simulink model "SixDOFSim"  (R2020b)
settings: Solver=VariableStepAuto  StartTime=0.0  StopTime=80  RelTol=1e-3
values from neighbouring files (symbols this model uses):
  A = sys_ol.A    [cost_condition_number.m]    (also in cost_coupling_control.m; cost_filter.m; coupling_control_scratch.m = sys.A; coupling_control_scratch2.m = sys.A)
  B = sys_ol.B    [cost_condition_number.m]    (also in cost_coupling_control.m; cost_filter.m; coupling_control_scratch.m = sys.B; coupling_control_scratch2.m = sys.B)
  C_tilde = zeros(size(C,1), size(A,1))    [SixDOFModel.m]    (also in cost_condition_number.m = struct_cond.C_tilde; cost_coupling_control.m = struct_cond.C_tilde; cost_filter.m = struct_cond.C_tilde; coupling_controller.m = T*C_resort)
  deltaX_init = Tx\deltaX_init    [SixDOFModel.m]    (also in coupling_controller_main.m = X_init-X_ap_simulink)
  eta_max = 15*pi/180    (= 0.261799387799)    [SixDOFModel.m]    (also in coupling_controller_main.m = 0.174532925199; load_messung_one_massmodel.m = 0.174532925199)
  eta_min = - 30*pi/180    (= -0.523598775598)    [SixDOFModel.m]    (also in coupling_controller_main.m = -0.436332312999; load_messung_one_massmodel.m = -0.436332312999)
  F = real(F)    [coupling_control_scratch.m]    (also in coupling_control_scratch2.m; coupling_controller.m = Kopt{end}; coupling_controller_main.m = -inv(C*(Ak\B)); coupling_controller_philipp.m = -inv(C*(Ak\B)))
  F_mod = F_ent(:,1:p/2)    [SixDOFModel.m]    (also in coupling_controller_main.m = F1*Q_mod; coupling_controller_philipp.m = F1*Q_mod; script_kein_theta_verk.m = F1*Q_mod)
  K_coupling = inv(Dstar)*compR    [SixDOFModel.m]    (also in coupling_controller_main.m = Kopt{1}; coupling_controller_philipp.m = Kopt{1}; script_kein_theta_verk.m = Kopt{1})
  latlon_init = [0;0]    [SixDOFModel.m]    (also in create_multi_model.m)
  m = i-1    [coupling_control_scratch.m]    (also in coupling_control_scratch2.m; defineABC.m = size(B_1,2) + size(B_2,2); implicit_linmod.m = length(U_ap); initializeParameters.m = 120000)
  noise_weight = [10 10 10 1 1 1 1 1 10 10 10 10 1 1 1 1 1 10]'    [SixDOFModel.m]
  P_e_init_1 = [0;0;-h_init_1]    [SixDOFModel.m]    (also in create_multi_model.m)
  P_e_init_2 = [0;0;-h_init_2]    [SixDOFModel.m]    (also in create_multi_model.m)
  q = X(5)    [nonlinear_6DOF.m]    (also in normieren.m = size (C,1))
  r = 5    [coupling_controller.m]    (also in coupling_controller_main.m = 100; coupling_controller_philipp.m = 200; nonlinear_6DOF.m = X(6); polgebiet.m = a2)
  sigmaf_max = 20*pi/180    (= 0.349065850399)    [SixDOFModel.m]    (also in coupling_controller_main.m; load_messung_one_massmodel.m)
  sigmaf_min = 0.5*pi/180    (= 0.00872664625997)    [SixDOFModel.m]    (also in coupling_controller_main.m; load_messung_one_massmodel.m)
  Tu = eye(size(B,2))    [SixDOFModel.m]    (also in normieren.m = zeros(p,p))
  Tx = eye(n)    [SixDOFModel.m]    (also in normieren.m = diag([200 15 50 0.1 0.1 0.1 45*pi/180 45*pi/180 10000 200 15)
  Ty = eye(size(C,1))    [SixDOFModel.m]    (also in normieren.m = zeros(q,q))
  U_ap = Tu\U_ap    [SixDOFModel.m]    (also in coupling_controller_main.m = AP(1,1).U_ap; create_multi_model.m = [U_ap_1;U_ap_2]; fsolve_trim.m = ap(11:14); trimValues.m = Z_ap(11:14))
  W_ap = W_ap(1:4)    [SixDOFModel.m]    (also in coupling_controller_philipp.m = (C*X_ap_simulink)')
  X_ap = [X_ap_1;X_ap_2]    [SixDOFModel.m]    (also in coupling_controller_main.m = AP(1,1).X_ap; create_multi_model.m; fsolve_trim.m = ap(1:10); trimValues.m = Z_ap(1:10))
  X_ap_simulink = Tx\X_ap_simulink    [SixDOFModel.m]    (also in coupling_controller_main.m = AP(1,1).X_ap_simulink; create_multi_model.m = [X_ap(1:8);X_ap(10);X_ap(11:18);X_ap(20)])
  X_init = Tx\X_init    [SixDOFModel.m]    (also in cost_coupling_control.m = struct_cond.X_init; cost_filter.m = struct_cond.X_init; coupling_controller_main.m = X_ap_simulink; create_multi_model.m = [X_init_1; X_init_2])
  xi_max = 25*pi/180    (= 0.436332312999)    [SixDOFModel.m]    (also in coupling_controller_main.m; load_messung_one_massmodel.m)
  xi_min = - xi_max    (= -0.436332312999)    [SixDOFModel.m]    (also in coupling_controller_main.m; load_messung_one_massmodel.m)
  zita_max = 30*pi/180    (= 0.523598775598)    [SixDOFModel.m]    (also in coupling_controller_main.m; load_messung_one_massmodel.m)
  zita_min = - zita_max    (= -0.523598775598)    [SixDOFModel.m]    (also in coupling_controller_main.m; load_messung_one_massmodel.m)
undefined symbols (not defined in the file or in its folder): Earth, globalParameters, Light, MIL, WGS84
libraries: aerolibfltsims x24, aerolibtransform2 x4, aerolibwind2 x4, simulink x3, shared6dof x1, aerolibanim x1
(part 1 of 3)
settings Model: Creator=teteu  LastModifiedBy=Markus
settings SolverCC: ZeroCrossAlgorithm=Adaptive
settings DebuggingCC: IgnoredZcDiagnostic=none  UnderSpecifiedDimensionMsg=warning

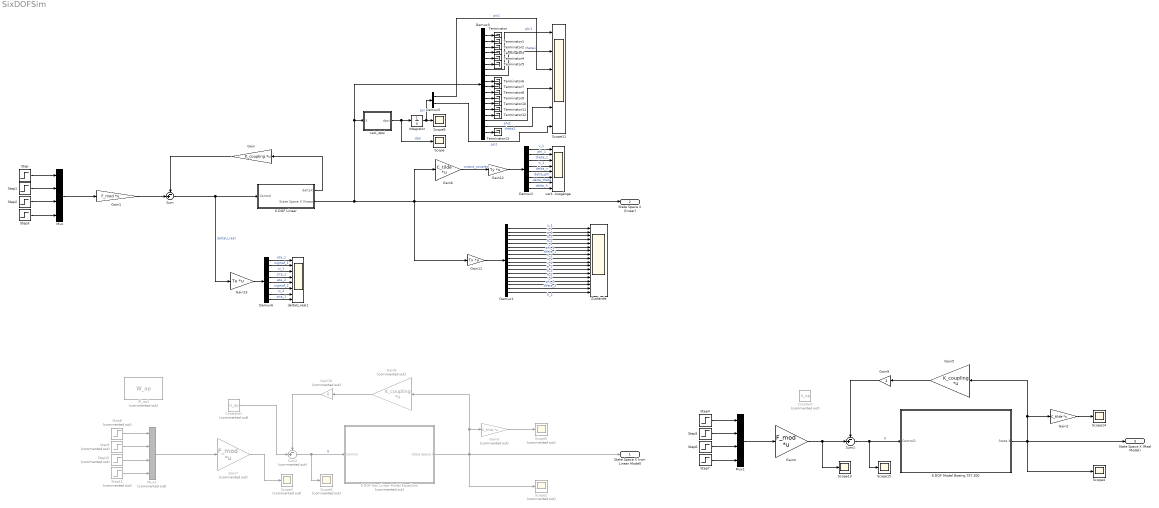
== system SixDOFSim ==
  6 DOF Linear : Subsystem
  6 DOF Model Boeing 757 200 : Subsystem
      mask Display: image('Eastern_Airlines_Boeing_757-225_N523EA_March_1990_DCW_4974892113-624x422.jpg'); % Use "Edit Image" on toolstrip to change.
  6 DOF Non Linear Model Equations : Subsystem  Commented=on
      mask Display: image('491461_1_En_8_Fig2_HTML.png');
  Constant : Constant  Commented=on  Value=U_ap
  Constant1 : Constant  Commented=on  Value=U_ap
  Demux1 : Demux  Outputs=18
  Demux2 : Demux  Outputs=8
  Demux3 : Demux  Outputs=18
  Demux5 : Demux  Outputs=2
  Demux6 : Demux  Outputs=8
  Gain : Gain  Gain=K_coupling  Multiplication=Matrix(K*u)
  Gain1 : Gain  Gain=F_mod  Multiplication=Matrix(K*u)
  Gain10 : Gain  Commented=on  Gain=0
  Gain11 : Gain  Gain=Tx  Multiplication=Matrix(K*u)
  Gain12 : Gain  Gain=Ty  Multiplication=Matrix(K*u)
  Gain13 : Gain  Gain=Tu  Multiplication=Matrix(K*u)
  Gain2 : Gain  Gain=C_tilde  Multiplication=Matrix(K*u)
  Gain3 : Gain  Commented=on  Gain=C_tilde  Multiplication=Matrix(K*u)
  Gain4 : Gain  Gain=F_mod  Multiplication=Matrix(K*u)
  Gain5 : Gain  Gain=K_coupling  Multiplication=Matrix(K*u)
  Gain6 : Gain  Gain=C_tilde  Multiplication=Matrix(K*u)
  Gain7 : Gain  Commented=on  Gain=F_mod  Multiplication=Matrix(K*u)
  Gain8 : Gain  Commented=on  Gain=K_coupling  Multiplication=Matrix(K*u)
  Gain9 : Gain
  Integrator : Integrator
  Mux : Mux
  Mux1 : Mux
  Mux2 : Mux  Commented=on
  Scope{,4,9,13..15} (6 alike) : Scope
  Scope11 : Scope  NumInputPorts=6
  Scope{2..3,5..6} (4 alike) : Scope  Commented=on
  Step{,1..3,5} (5 alike) : Step  Time=10  After=0  SampleTime=0
  Step10 : Step  Commented=on  Time=10  After=0  SampleTime=0
  Step11 : Step  Commented=on  Time=10  SampleTime=0
  Step4 : Step  Time=0  After=0  SampleTime=0
  Step6 : Step  Time=0  After=-0.0734  SampleTime=0
  Step7 : Step  Time=0  After=5000  SampleTime=0
  Step8 : Step  Commented=on  Time=10  After=0  SampleTime=0
  Step9 : Step  Commented=on  Time=10  After=0  SampleTime=0
  Sum : Sum  Inputs=-+|
  Sum1 : Sum  Inputs=-+|
  Sum2 : Sum  Commented=on  Inputs=-+|
  Terminator{,1..13} (14 alike) : Terminator
  W_ap1 : Constant  Commented=on  Value=W_ap
  Zustände : Scope  NumInputPorts=18
  calc_dpsi : MATLAB Function  TreatAsAtomicUnit=on
  deltaU_real1 : Scope  NumInputPorts=8
  verk. Ausgänge : Scope  NumInputPorts=8
  State Space X (non Linear Model) : Outport
  State Space X (linear) : Outport  Port=2
  State Space X (Real Model) : Outport  Port=3
  wires:
  Gain/1 -> Sum/1
  6 DOF Non Linear Model Equations/1(State Space X) -> Gain8/1, Gain3/1, State Space X (non Linear Model)/1, Scope2/1
  Mux/1 -> Gain1/1
  Gain1/1 -> Sum/2
  6 DOF Linear/1(deltaX) -> Gain/1
  Gain3/1 -> Scope5/1
  Gain6/1 -> Gain12/1  "output_coupled"
  Sum2/1 -> Scope6/1, 6 DOF Non Linear Model Equations/1(Control)  "U"
  Gain8/1 -> Gain10/1
  Gain7/1 -> Scope3/1
  Mux2/1 -> Gain7/1
  Demux1/1 -> Zustände/1  "u_1"
  Demux1/2 -> Zustände/2  "v_1"
  Demux1/3 -> Zustände/3  "w_1"
  Demux1/4 -> Zustände/4  "p_1"
  Demux1/5 -> Zustände/5  "q_1"
  Demux1/6 -> Zustände/6  "r_1"
  Demux1/7 -> Zustände/7  "phi_1"
  Demux1/8 -> Zustände/8  "theta_1"
  Demux1/9 -> Zustände/9  "h_1"
  Demux1/10 -> Zustände/10  "u_2"
  Demux1/11 -> Zustände/11  "v_2"
  Demux1/12 -> Zustände/12  "w_2"
  Demux1/13 -> Zustände/13  "p_2"
  Demux1/14 -> Zustände/14  "q_2"
  Demux1/15 -> Zustände/15  "r_2"
  Demux1/16 -> Zustände/16  "phi_2"
  Demux2/8 -> verk. Ausgänge/8  "delta_h"
  Demux2/7 -> verk. Ausgänge/7  "delta_theta"
  Demux2/6 -> verk. Ausgänge/6  "delta_phi"
  Demux2/3 -> verk. Ausgänge/3  "theta_1"
  Demux2/2 -> verk. Ausgänge/2  "phi_1"
  Demux2/4 -> verk. Ausgänge/4  "h_1"
  Demux2/5 -> verk. Ausgänge/5  "delta_v"
  Demux2/1 -> verk. Ausgänge/1  "v_1"
  calc_dpsi/1(dpsi) -> Scope/1, Integrator/1  "dpsi"
  Integrator/1 -> Demux5/1, Scope9/1  "psi"
  Demux3/1 -> Terminator/1
  Demux3/2 -> Terminator1/1
  Demux3/3 -> Terminator2/1
  Demux3/4 -> Terminator3/1
  Demux3/5 -> Terminator4/1
  Demux3/6 -> Terminator5/1
  Demux3/7 -> Scope11/1  "phi1"
  Demux3/8 -> Scope11/2  "theta1"
  Demux3/10 -> Terminator7/1
  Demux3/11 -> Terminator8/1
  Demux3/12 -> Terminator9/1
  Demux3/13 -> Terminator10/1
  Demux3/14 -> Terminator11/1
  Demux3/16 -> Scope11/4  "phi2"
  Demux5/1 -> Scope11/3  "psi1"
  Demux5/2 -> Scope11/6  "psi2"
  6 DOF Linear/2(State Space X (linear)) -> Demux3/1, calc_dpsi/1(X), State Space X (linear)/1, Gain11/1, Gain6/1
  Demux1/18 -> Zustände/18  "h_2"
  Demux1/17 -> Zustände/17  "theta_2"
  Demux3/9 -> Terminator6/1
  Demux3/15 -> Terminator12/1
  Demux3/17 -> Scope11/5  "theta2"
  Demux3/18 -> Terminator13/1
  Step/1 -> Mux/1
  Step1/1 -> Mux/2
  Step2/1 -> Mux/3
  Step3/1 -> Mux/4
  Sum1/1 -> 6 DOF Model Boeing 757 200/1(Control1), Scope15/1  "U"
  Gain4/1 -> Sum1/2, Scope13/1
  6 DOF Model Boeing 757 200/1(State X) -> State Space X (Real Model)/1, Gain5/1, Gain2/1, Scope4/1
  Gain2/1 -> Scope14/1
  Gain5/1 -> Gain9/1
  Step7/1 -> Mux1/4
  Step6/1 -> Mux1/3
  Step4/1 -> Mux1/1
  Step5/1 -> Mux1/2
  Mux1/1 -> Gain4/1
  Step11/1 -> Mux2/4
  Step10/1 -> Mux2/3
  Step8/1 -> Mux2/1
  Step9/1 -> Mux2/2
  Gain9/1 -> Sum1/1
  Gain10/1 -> Sum2/1
  Constant1/1 -> Sum2/2
  Gain11/1 -> Demux1/1
  Gain12/1 -> Demux2/1
  Demux6/4 -> deltaU_real1/4  "zita_1"
  Demux6/3 -> deltaU_real1/3  "xi_1"
  Demux6/7 -> deltaU_real1/7  "xi_2"
  Demux6/6 -> deltaU_real1/6  "sigmaf_2"
  Demux6/1 -> deltaU_real1/1  "eta_1"
  Demux6/2 -> deltaU_real1/2  "sigmaf_1"
  Demux6/5 -> deltaU_real1/5  "eta_2"
  Sum/1 -> Gain13/1, 6 DOF Linear/1(Control)  "deltaU_real"
  Demux6/8 -> deltaU_real1/8  "zita_2"
  Gain13/1 -> Demux6/1

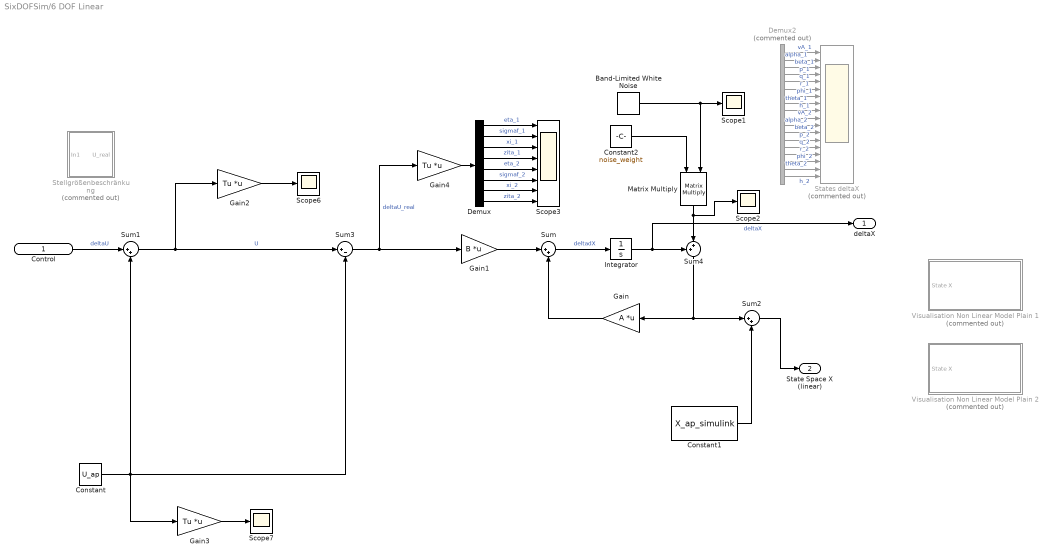
== system SixDOFSim/6 DOF Linear ==
  Control : Inport
  Band-Limited White Noise : simulink/Sources/Band-Limited White Noise  Cov=[0.0]  Ts=0.01  seed=[23341]
  Constant : Constant  Value=U_ap
  Constant1 : Constant  Value=X_ap_simulink
  Constant2 : Constant  Value=noise_weight
  Demux : Demux  Outputs=8
  Demux2 : Demux  Commented=on  Outputs=18
  Gain : Gain  Gain=A  Multiplication=Matrix(K*u)
  Gain1 : Gain  Gain=B  Multiplication=Matrix(K*u)
  Gain2 : Gain  Gain=Tu  Multiplication=Matrix(K*u)
  Gain3 : Gain  Gain=Tu  Multiplication=Matrix(K*u)
  Gain4 : Gain  Gain=Tu  Multiplication=Matrix(K*u)
  Integrator : Integrator  InitialCondition=deltaX_init
  Matrix Multiply : Product  Multiplication=Matrix(*)
  Scope{1..2,6..7} (4 alike) : Scope
  Scope3 : Scope  NumInputPorts=8
  States deltaX : Scope  Commented=on  NumInputPorts=18
  Stellgrößenbeschränkung : Subsystem  Commented=on
  Sum : Sum  Inputs=|++
  Sum1 : Sum  Inputs=|++
  Sum2 : Sum  Inputs=|++
  Sum3 : Sum  Inputs=|+-
  Sum4 : Sum  Inputs=++|
  Visualisation Non Linear Model Plain 1 : Subsystem  Commented=on
  Visualisation Non Linear Model Plain 2 : Subsystem  Commented=on
  deltaX : Outport
  State Space X (linear) : Outport  Port=2
  wires:
  Gain1/1 -> Sum/1
  Sum/1 -> Integrator/1  "deltadX"
  Gain/1 -> Sum/2
  Control/1 -> Sum1/1  "deltaU"
  Constant/1 -> Gain3/1, Sum1/2, Sum3/2
  Sum1/1 -> Sum3/1, Gain2/1  "U"
  Sum2/1 -> State Space X (linear)/1
  Constant1/1 -> Sum2/2
  Sum3/1 -> Gain4/1, Gain1/1  "deltaU_real"
  Demux/1 -> Scope3/1  "eta_1"
  Demux/2 -> Scope3/2  "sigmaf_1"
  Demux/3 -> Scope3/3  "xi_1"
  Demux/4 -> Scope3/4  "zita_1"
  Demux/5 -> Scope3/5  "eta_2"
  Demux/6 -> Scope3/6  "sigmaf_2"
  Demux/7 -> Scope3/7  "xi_2"
  Demux/8 -> Scope3/8  "zita_2"
  Demux2/9 -> States deltaX/9  "h_1"
  Demux2/13 -> States deltaX/13  "p_2"
  Demux2/6 -> States deltaX/6  "r_1"
  Demux2/15 -> States deltaX/15  "r_2"
  Demux2/18 -> States deltaX/18  "h_2"
  Demux2/14 -> States deltaX/14  "q_2"
  Demux2/8 -> States deltaX/8  "theta_1"
  Demux2/17 -> States deltaX/17  "theta_2"
  Demux2/11 -> States deltaX/11  "alpha_2"
  Demux2/2 -> States deltaX/2  "alpha_1"
  Demux2/3 -> States deltaX/3  "beta_1"
  Demux2/1 -> States deltaX/1  "vA_1"
  Demux2/16 -> States deltaX/16  "phi_2"
  Demux2/12 -> States deltaX/12  "beta_2"
  Demux2/4 -> States deltaX/4  "p_1"
  Demux2/7 -> States deltaX/7  "phi_1"
  Demux2/5 -> States deltaX/5  "q_1"
  Demux2/10 -> States deltaX/10  "vA_2"
  Integrator/1 -> deltaX/1, Sum4/1  "deltaX"
  Sum4/1 -> Sum2/1, Gain/1
  Band-Limited White Noise/1 -> Matrix Multiply/2, Scope1/1
  Constant2/1 -> Matrix Multiply/1
  Matrix Multiply/1 -> Sum4/2, Scope2/1
  Gain2/1 -> Scope6/1
  Gain3/1 -> Scope7/1
  Gain4/1 -> Demux/1

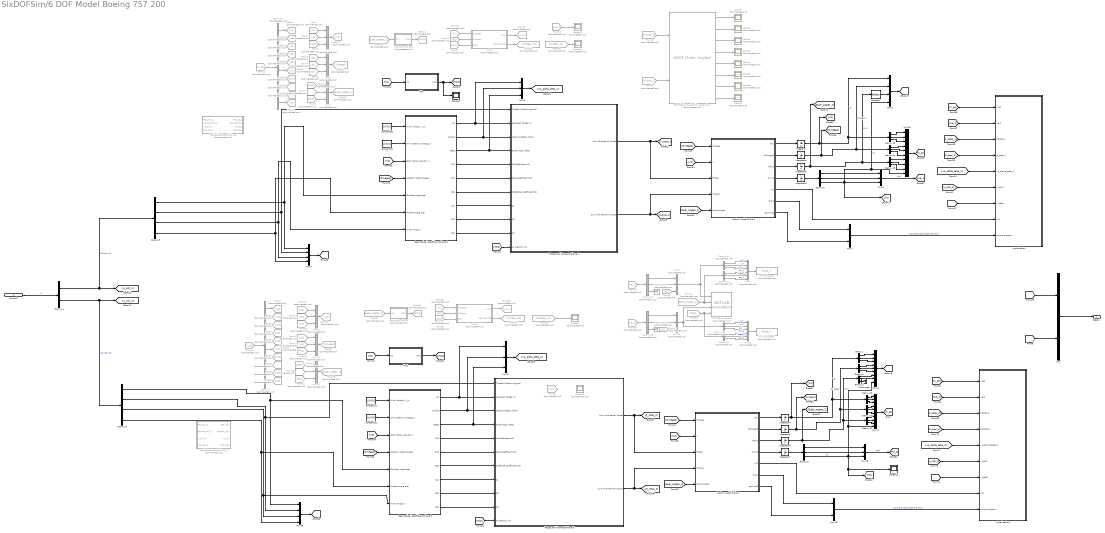
== system SixDOFSim/6 DOF Model Boeing 757 200 ==
  Control1 : Inport
  6DOF (Euler Angles) for comparison : shared6dof/6DOF (Euler Angles)  Commented=on  units=Metric (MKS)  mtype=Fixed  rep=Euler Angles  xme_0=[0 0 0]  Vm_0=[0 0 0]  eul_0=[0 0 0]  pm_0=[0 0 0]  mass_0=1.0  mass_e=0.5  mass_f=2.0  inertia=eye(3)  inertia_e=eye(3)  inertia_f=2*eye(3)  k_quat=1.0  vre_flag=on  abi_flag=off  aMode=0  xme_statename=''  Vm_statename=''  eul_statename=''  quat_statename=''  pm_statename=''  mass_statename=''
      settings: SourceProductBaseCode=AE,PW,MT,UV,VE,VP
  Constant{21..22,30..31} (4 alike) : Constant  Value=[0 0 0]
  Demux{,1..2,6,9..15} (11 alike) : Demux  Outputs=3
  Demux{16..21} (6 alike) : Demux  Commented=on  Outputs=3
  Demux3 : Demux  Commented=on  Outputs=10
  Demux4 : Demux  Outputs=2
  Demux5 : Demux
  Demux7 : Demux  Commented=on  Outputs=10
  Demux8 : Demux
  Forces and Moments Plane 2 : Subsystem
  Forces and Moments Plane 3 : Subsystem
  From : From  Commented=on  GotoTag=u1
  From1 : From  Commented=on  GotoTag=v1
  From10 : From  Commented=on  GotoTag=F_total_2
  From11 : From  Commented=on  GotoTag=M_total_2
  From12 : From  Commented=on  GotoTag=X_g1
  From13 : From  Commented=on  GotoTag=u2
  From14 : From  Commented=on  GotoTag=v2
  From15 : From  Commented=on  GotoTag=w2
  From16 : From  Commented=on  GotoTag=p2
  From17 : From  Commented=on  GotoTag=q2
  From18 : From  Commented=on  GotoTag=r2
  From19 : From  Commented=on  GotoTag=phi2
  From2 : From  Commented=on  GotoTag=w1
  From20 : From  Commented=on  GotoTag=theta2
  From21 : From  Commented=on  GotoTag=psi2
  From24 : From  Commented=on  GotoTag=h1
  From25 : From  Commented=on  GotoTag=omega_w1
  From26 : From  Commented=on  GotoTag=Euler_angles_1
  From27 : From  Commented=on  GotoTag=DCM1
  From28 : From  Commented=on  GotoTag=V1
  From29 : From  Commented=on  GotoTag=V_w1
  From3 : From  Commented=on  GotoTag=p1
  From4 : From  Commented=on  GotoTag=q1
  From43 : From  Commented=on  GotoTag=X_g2
  From44 : From  Commented=on  GotoTag=Euler_angles_1
  From45 : From  Commented=on  GotoTag=h1
  From47 : From  Commented=on  GotoTag=h2
  From48 : From  Commented=on  GotoTag=Xe_2
  From49 : From  Commented=on  GotoTag=Xe_1
  From5 : From  Commented=on  GotoTag=r1
  From50 : From  Commented=on  GotoTag=Phi2
  From55 : From  Commented=on  GotoTag=h2
  From56 : From  Commented=on  GotoTag=omega_w2
  From57 : From  Commented=on  GotoTag=Euler_angles_2
  From58 : From  Commented=on  GotoTag=DCM2
  From59 : From  Commented=on  GotoTag=V2
  From6 : From  Commented=on  GotoTag=phi1
  From60 : From  Commented=on  GotoTag=V_w2
  From7 : From  Commented=on  GotoTag=theta1
  From8 : From  Commented=on  GotoTag=psi1
  Geometrical Coefficients Plane 2 : Subsystem
  Geometrical Coefficients Plane 3 : Subsystem
  Goto1 : Goto  Commented=on  GotoTag=u2
  Goto10 : Goto  Commented=on  GotoTag=h2
  Goto11 : Goto  Commented=on  GotoTag=V2
  Goto12 : Goto  Commented=on  GotoTag=u1
  Goto13 : Goto  Commented=on  GotoTag=v1
  Goto14 : Goto  Commented=on  GotoTag=w1
  Goto15 : Goto  Commented=on  GotoTag=p1
  Goto16 : Goto  Commented=on  GotoTag=q1
  Goto17 : Goto  Commented=on  GotoTag=r1
  Goto18 : Goto  Commented=on  GotoTag=phi1
  Goto19 : Goto  Commented=on  GotoTag=theta1
  Goto2 : Goto  Commented=on  GotoTag=v2
  Goto20 : Goto  Commented=on  GotoTag=psi1
  Goto21 : Goto  Commented=on  GotoTag=h1
  Goto24 : Goto  Commented=on  GotoTag=V1
  Goto25 : Goto  Commented=on  GotoTag=Omega1
  Goto26 : Goto  Commented=on  GotoTag=Euler_angles_1
  Goto27 : Goto  Commented=on  GotoTag=DCM1
  Goto28 : Goto  Commented=on  GotoTag=V_w1
  Goto29 : Goto  Commented=on  GotoTag=omega_w1
  Goto3 : Goto  Commented=on  GotoTag=w2
  Goto37 : Goto  Commented=on  GotoTag=Omega2
  Goto38 : Goto  Commented=on  GotoTag=Euler_angles_2
  Goto4 : Goto  Commented=on  GotoTag=p2
  Goto5 : Goto  Commented=on  GotoTag=q2
  Goto52 : Goto  Commented=on  GotoTag=DCM2
  Goto53 : Goto  Commented=on  GotoTag=V_w2
  Goto54 : Goto  Commented=on  GotoTag=omega_w2
  Goto6 : Goto  Commented=on  GotoTag=r2
  Goto7 : Goto  Commented=on  GotoTag=phi2
  Goto8 : Goto  Commented=on  GotoTag=theta2
  Goto9 : Goto  Commented=on  GotoTag=psi2
  Integrator : Integrator  InitialCondition=X_init(1:3)
  Integrator1 : Integrator  InitialCondition=X_init(4:6)
  Integrator2 : Integrator  InitialCondition=[X_init(7:8);X_ap(9)]
  Integrator3 : Integrator  InitialCondition=[0; 0; X_init(9)]
  Integrator4 : Integrator  InitialCondition=X_init(10:12)
  Integrator5 : Integrator  InitialCondition=X_init(13:15)
  Integrator6 : Integrator  InitialCondition=[X_init(16:17);X_ap(19)]
  Integrator7 : Integrator  InitialCondition=[0; 0; X_init(18)]
  MATLAB Animation : aerolibanim/MATLAB Animation  Tag=Matlab Animation 6 DOF  Commented=on  Vehicles=2  Geometries={ 'astredwedge.mat', 'astredwedge.mat'}  BoundingBoxCoordinates=[-500,500,-500,500,-500,500]  CameraOffset=[-100,50,-50]  CameraViewAngle=20  SampleTime=0.2  FigurePosition=[1921,138,1536,774]
      settings: SourceProductBaseCode=AE
  MATLAB Function3 : MATLAB Function  Commented=on  TreatAsAtomicUnit=on
  MATLAB Function4 : MATLAB Function  Commented=on  TreatAsAtomicUnit=on
  Motion model Plain3 : Subsystem
  Motion model Plane 2 : Subsystem
  Mux : Mux  Inputs=2
  Mux{1..4,12..14,20} (8 alike) : Mux  Commented=on  Inputs=3
  Mux10 : Mux  Inputs=9
  Mux11 : Mux  Inputs=10
  Mux{6,8,15,17} (4 alike) : Mux  Inputs=3
  Mux16 : Mux  Inputs=2
  Mux18 : Mux
  Mux19 : Mux  Inputs=10
  Mux21 : Mux  Commented=on  Inputs=6
  Mux22 : Mux  Commented=on  Inputs=6
  Mux5 : Mux
  Mux7 : Mux  Inputs=2
  Mux9 : Mux
  Rho : Subsystem
  Rho1 : Subsystem
  Scope{,1..7,13..16} (12 alike) : Scope  Commented=on
  Scope12 : Scope
  Scope17 : Scope
  Selector : Selector  InputPortWidth=3  IndexOptions=Index vector (dialog)  Indices=[1 2]  OutputSizes=1
  Stellgrößenbeschränkung : Subsystem  Commented=on
  Stellgrößenbeschränkung 2 : Subsystem  Commented=on
  Terminator : Terminator
  Terminator1 : Terminator  Commented=on
  Terminator2 : Terminator  Commented=on
  To Workspace : ToWorkspace  Commented=on  VariableName=Plane_1  SaveFormat=Timeseries  SampleTime=-1
  To Workspace1 : ToWorkspace  Commented=on  VariableName=Plane_2  SaveFormat=Timeseries  SampleTime=-1
  Visualization : Subsystem
  Visualization1 : Subsystem
  Wind : Subsystem  Commented=on
  Wind1 : Subsystem  Commented=on
  State X : Outport
  wires:
  From12/1 -> Demux3/1
  Demux3/1 -> Goto12/1
  Demux3/2 -> Goto13/1
  Demux3/3 -> Goto14/1
  Demux3/4 -> Goto15/1
  Demux3/5 -> Goto16/1
  Demux3/6 -> Goto17/1
  Demux3/7 -> Goto18/1
  Demux3/8 -> Goto19/1
  Demux3/9 -> Goto20/1
  Demux3/10 -> Goto21/1
  Demux4/1 -> [u_soll_1], Demux5/1  "Control p1"
  Control1/1 -> Demux4/1  "U"
  From2/1 -> Mux1/3
  Mux1/1 -> Goto24/1
  From1/1 -> Mux1/2
  From/1 -> Mux1/1
  From3/1 -> Mux2/1
  From4/1 -> Mux2/2
  Mux2/1 -> Goto25/1
  From5/1 -> Mux2/3
  From8/1 -> Mux3/3
  Mux3/1 -> Goto26/1
  From7/1 -> Mux3/2
  From6/1 -> Mux3/1
  [Omega1] -> Geometrical Coefficients Plane 2/4(Rotation rates Omega)
  [V1] -> Geometrical Coefficients Plane 2/3(Body frame velocity V)
  MATLAB Function3/1(DCM) -> Goto27/1
  From26/1 -> MATLAB Function3/1(Phi)
  From28/1 -> Wind/1(Airspeed)
  From24/1 -> Wind/2(Altitude)
  From27/1 -> Wind/3(DCM)
  Wind/1(V_w1) -> Goto28/1
  Wind/2(pg1,qg1,rg1) -> Goto29/1
  [h1] -> Rho/1(h1)
  Rho/1(rho1) -> Scope17/1, [rho1]
  Geometrical Coefficients Plane 2/7(CL1) -> Forces and Moments Plane 2/8(CL)
  Geometrical Coefficients Plane 2/8(CM1) -> Forces and Moments Plane 2/9(CM)
  Geometrical Coefficients Plane 2/9(CN1) -> Forces and Moments Plane 2/10(CN)
  Geometrical Coefficients Plane 2/2(alpha1) -> Mux8/2, Forces and Moments Plane 2/3(Angle of Attack Alpha)
  Geometrical Coefficients Plane 2/3(beta1) -> Mux8/3, Forces and Moments Plane 2/4(Slide Angle  beta)
  Geometrical Coefficients Plane 2/1(vA1) -> Mux8/1, Forces and Moments Plane 2/2(Approach speed vA)
  Geometrical Coefficients Plane 2/4(CA1) -> Forces and Moments Plane 2/5(Lift Coeficcient CA)
  Geometrical Coefficients Plane 2/5(CW1) -> Forces and Moments Plane 2/6(Drag Coefficient CW)
  Geometrical Coefficients Plane 2/6(CQ1) -> Forces and Moments Plane 2/7(Sideforce Coefficient CQ)
  [rho1] -> Forces and Moments Plane 2/11(Air Density rho)
  Forces and Moments Plane 2/1(Sum of external Forces) -> Motion model Plane 2/3(Forces), [F_total_1]
  Forces and Moments Plane 2/2(Sum of external Torques) -> Motion model Plane 2/4(Torque), [M_total_1]
  [Euler_angles_1] -> Motion model Plane 2/5(Euler angles)
  [Omega1] -> Motion model Plane 2/1(Omega)
  [V1] -> Motion model Plane 2/2(V)
  Motion model Plane 2/1(dV1) -> Integrator/1
  Motion model Plane 2/2(dOmega1) -> Integrator1/1
  Motion model Plane 2/3(dPhi1) -> Integrator2/1
  Integrator2/1 -> [Euler_angles_1], Selector/1, Demux15/1  "Phi1"
  Integrator1/1 -> [Omega1], Mux5/2, Demux14/1  "Omega1"
  Integrator/1 -> [V1], Mux5/1, Demux13/1  "V1"
  Motion model Plane 2/4(dxyh1) -> Integrator3/1
  Integrator3/1 -> Demux6/1
  Demux6/2 -> Mux6/2
  Demux6/1 -> Mux6/1
  Selector/1 -> Mux5/3
  Mux5/1 -> [X_red1]
  Mux6/1 -> [Xe_1]  "Xe1"
  [X_red1] -> Mux/1
  [X_g1] -> Visualization/1(X_g1)
  [Xe_1] -> Visualization/2(Xe_1)
  Motion model Plane 2/6(chsi1) -> Mux7/1
  Motion model Plane 2/7(gamma1) -> Mux7/2
  Mux7/1 -> Visualization/9(cource angles 1)  "Course angles (gamma,chsi)"
  [F_total_1] -> Visualization/3(F_total_1)
  [M_total_1] -> Visualization/4(M_total_1)
  Mux8/1 -> [vA_alpha_beta_1]
  [vA_alpha_beta_1] -> Visualization/5(vA_alpha_beta_1)
  Motion model Plane 2/5(vk1) -> Visualization/8(vk1)
  Mux9/1 -> [u_stell1]
  [u_soll_1] -> Visualization/6(u_soll1)
  [u_stell1] -> Visualization/7(u_stell1)
  [u_stell2] -> Visualization1/7(u_stell2)
  [u_soll_2] -> Visualization1/6(u_soll2)
  Mux18/1 -> [u_stell2]
  Motion model Plain3/5(vk2) -> Visualization1/8(vk2)
  [vA_alpha_beta_2] -> Visualization1/5(vA_alpha_beta_2)
  Mux17/1 -> [vA_alpha_beta_2]
  [M_total_2] -> Visualization1/4(M_total_2)
  [F_total_2] -> Visualization1/3(F_total_2)
  Mux16/1 -> Visualization1/9(course angles 2)  "Course angles (gamma,chsi)"
  Motion model Plain3/7(gamma2) -> Mux16/2
  Motion model Plain3/6(chsi2) -> Mux16/1
  [Xe_2] -> Visualization1/2(Xe_2)
  [X_g2] -> Visualization1/1(X_g2)
  Mux15/1 -> [Xe_2]  "Xe_2"
  Mux10/1 -> [X_red2]
  Demux9/1 -> Mux15/1
  Demux9/2 -> Mux15/2
  Demux9/3 -> Mux10/9, Mux11/10, Mux15/3, [h2], Scope12/1  "h2"
  Integrator7/1 -> Demux9/1
  Motion model Plain3/4(dxyh2) -> Integrator7/1
  Integrator5/1 -> Demux1/1, Demux11/1, [Omega2]  "Omega2"
  Integrator6/1 -> [Euler_angles_2], Demux12/1, Demux2/1  "Phi2"
  Motion model Plain3/3(dPhi2) -> Integrator6/1
  Motion model Plain3/2(dOmega2) -> Integrator5/1
  Motion model Plain3/1(dV2) -> Integrator4/1
  [V2] -> Motion model Plain3/2(V)
  [Omega2] -> Motion model Plain3/1(Omega)
  [Euler_angles_2] -> Motion model Plain3/5(Euler angles)
  Forces and Moments Plane 3/2(Sum of external Torques) -> Motion model Plain3/4(Torque), [M_total_2]
  Forces and Moments Plane 3/1(Sum of external Forces) -> Motion model Plain3/3(Forces), [F_total_2]
  [rho2] -> Forces and Moments Plane 3/11(Air Density rho)
  Geometrical Coefficients Plane 3/6(CQ2) -> Forces and Moments Plane 3/7(Sideforce Coefficient CQ)
  Geometrical Coefficients Plane 3/5(CW2) -> Forces and Moments Plane 3/6(Drag Coefficient CW)
  Geometrical Coefficients Plane 3/4(CA2) -> Forces and Moments Plane 3/5(Lift Coeficcient CA)
  Geometrical Coefficients Plane 3/1(vA2) -> Forces and Moments Plane 3/2(Approach speed vA), Mux17/1
  Geometrical Coefficients Plane 3/3(beta2) -> Forces and Moments Plane 3/4(Slide Angle  beta), Mux17/3
  Geometrical Coefficients Plane 3/2(alpha2) -> Forces and Moments Plane 3/3(Angle of Attack Alpha), Mux17/2
  Geometrical Coefficients Plane 3/9(CN2) -> Forces and Moments Plane 3/10(CN)
  Geometrical Coefficients Plane 3/8(CM2) -> Forces and Moments Plane 3/9(CM)
  Geometrical Coefficients Plane 3/7(CL2) -> Forces and Moments Plane 3/8(CL)
  Rho1/1(rho2) -> [rho2]
  [h2] -> Rho1/1(h2)
  Wind1/2(pg2,qg2,rg2) -> Goto54/1
  Wind1/1(V_w2) -> Goto53/1
  From58/1 -> Wind1/3(DCM)
  From55/1 -> Wind1/2(Altitude)
  From59/1 -> Wind1/1(Airspeed)
  From57/1 -> MATLAB Function4/1(Phi)
  MATLAB Function4/1(DCM) -> Goto52/1
  [V2] -> Geometrical Coefficients Plane 3/3(Body frame velocity V)
  [Omega2] -> Geometrical Coefficients Plane 3/4(Rotation rates Omega)
  Demux4/2 -> [u_soll_2], Demux8/1  "Control p2"
  Mux/1 -> State X/1
  [X_red2] -> Mux/2
  Demux/1 -> Mux10/1
  Demux/2 -> Mux10/2
  Demux/3 -> Mux10/3
  Demux1/1 -> Mux10/4
  Demux1/2 -> Mux10/5
  Demux1/3 -> Mux10/6
  Demux2/1 -> Mux10/7
  Demux2/2 -> Mux10/8
  Demux10/1 -> Mux11/1
  Demux11/3 -> Mux11/6
  Demux11/2 -> Mux11/5
  Mux11/1 -> [X_g2]
  Demux10/2 -> Mux11/2
  Integrator4/1 -> Demux/1, Demux10/1, [V2]  "V2"
  Demux12/1 -> Mux11/7
  Demux10/3 -> Mux11/3
  Demux11/1 -> Mux11/4
  Demux12/2 -> Mux11/8
  Demux12/3 -> Mux11/9
  Demux7/2 -> Goto2/1
  Demux7/5 -> Goto5/1
  Demux7/10 -> Goto10/1
  Demux7/8 -> Goto8/1
  Demux7/3 -> Goto3/1
  Demux7/6 -> Goto6/1
  Demux7/7 -> Goto7/1
  Demux7/1 -> Goto1/1
  Demux7/9 -> Goto9/1
  Demux7/4 -> Goto4/1
  From43/1 -> Demux7/1
  From13/1 -> Mux12/1
  From19/1 -> Mux14/1
  Mux12/1 -> Goto11/1
  From18/1 -> Mux13/3
  From14/1 -> Mux12/2
  From16/1 -> Mux13/1
  From20/1 -> Mux14/2
  Mux13/1 -> Goto37/1
  From17/1 -> Mux13/2
  Mux14/1 -> Goto38/1
  From21/1 -> Mux14/3
  From15/1 -> Mux12/3
  Demux2/3 -> Terminator/1
  Mux19/1 -> [X_g1]
  Demux13/3 -> Mux19/3
  Demux15/1 -> Mux19/7
  Demux14/1 -> Mux19/4
  Demux13/2 -> Mux19/2
  Demux14/2 -> Mux19/5
  Demux14/3 -> Mux19/6
  Demux15/2 -> Mux19/8
  Demux13/1 -> Mux19/1
  Demux15/3 -> Mux19/9
  From60/1 -> Scope13/1
  From56/1 -> Scope14/1
  Constant22/1 -> Geometrical Coefficients Plane 3/2(Wind rotation omega_w)
  Constant21/1 -> Geometrical Coefficients Plane 3/1(Wind velocity V_w)
  From29/1 -> Scope16/1
  From25/1 -> Scope15/1
  Constant30/1 -> Geometrical Coefficients Plane 2/1(Wind velocity V_w)
  Constant31/1 -> Geometrical Coefficients Plane 2/2(Wind rotation omega_w)
  6DOF (Euler Angles) for comparison/3 -> Scope2/1
  6DOF (Euler Angles) for comparison/5 -> Scope4/1
  From10/1 -> 6DOF (Euler Angles) for comparison/1
  6DOF (Euler Angles) for comparison/8 -> Scope7/1
  6DOF (Euler Angles) for comparison/6 -> Scope5/1
  6DOF (Euler Angles) for comparison/4 -> Scope3/1
  6DOF (Euler Angles) for comparison/2 -> Scope1/1
  From11/1 -> 6DOF (Euler Angles) for comparison/2
  6DOF (Euler Angles) for comparison/7 -> Scope6/1
  6DOF (Euler Angles) for comparison/1 -> Scope/1
  Demux6/3 -> [h1], Mux6/3, Mux5/4, Mux19/10  "h1"
  Demux17/3 -> Mux22/6  "psi_1"
  Demux18/1 -> Mux20/1
  Demux17/2 -> Mux22/5  "theta_1"
  From45/1 -> Mux4/3
  Demux19/1 -> Mux4/1
  Demux20/3 -> Mux21/3  "z_1"
  Demux18/2 -> Mux20/2
  Demux21/1 -> Mux21/4  "phi_1"
  Mux4/1 -> Demux20/1, MATLAB Animation/1
  Demux16/2 -> Mux22/2  "y_1"
  From47/1 -> Mux20/3
  Mux22/1 -> To Workspace1/1
  From48/1 -> Demux18/1
  Demux21/2 -> Mux21/5  "theta_1"
  Demux17/1 -> Mux22/4  "phi_1"
  Demux20/1 -> Mux21/1  "x_1"
  Mux21/1 -> To Workspace/1
  Demux16/1 -> Mux22/1  "x_1"
  Demux19/2 -> Mux4/2
  Mux20/1 -> MATLAB Animation/3, Demux16/1
  Demux20/2 -> Mux21/2  "y_1"
  From44/1 -> Demux21/1, MATLAB Animation/2
  Demux21/3 -> Mux21/6  "psi_1"
  Demux18/3 -> Terminator2/1
  Demux16/3 -> Mux22/3  "z_1"
  From49/1 -> Demux19/1
  Demux19/3 -> Terminator1/1
  From50/1 -> Demux17/1, MATLAB Animation/4
  Demux5/2 -> Forces and Moments Plane 2/1(Throttel Position sigmaf), Mux9/2
  Demux5/3 -> Geometrical Coefficients Plane 2/7(Airlon Angle xi), Mux9/3
  Demux5/1 -> Geometrical Coefficients Plane 2/5(Elevator Angle eta), Mux9/1
  Demux5/4 -> Geometrical Coefficients Plane 2/6(Rudder Angle zita), Mux9/4
  Demux8/4 -> Mux18/4, Geometrical Coefficients Plane 3/6(Rudder Angle zita)
  Demux8/1 -> Geometrical Coefficients Plane 3/5(Elevator Angle eta), Mux18/1
  Demux8/2 -> Forces and Moments Plane 3/1(Throttel Position sigmaf), Mux18/2
  Demux8/3 -> Mux18/3, Geometrical Coefficients Plane 3/7(Airlon Angle xi)

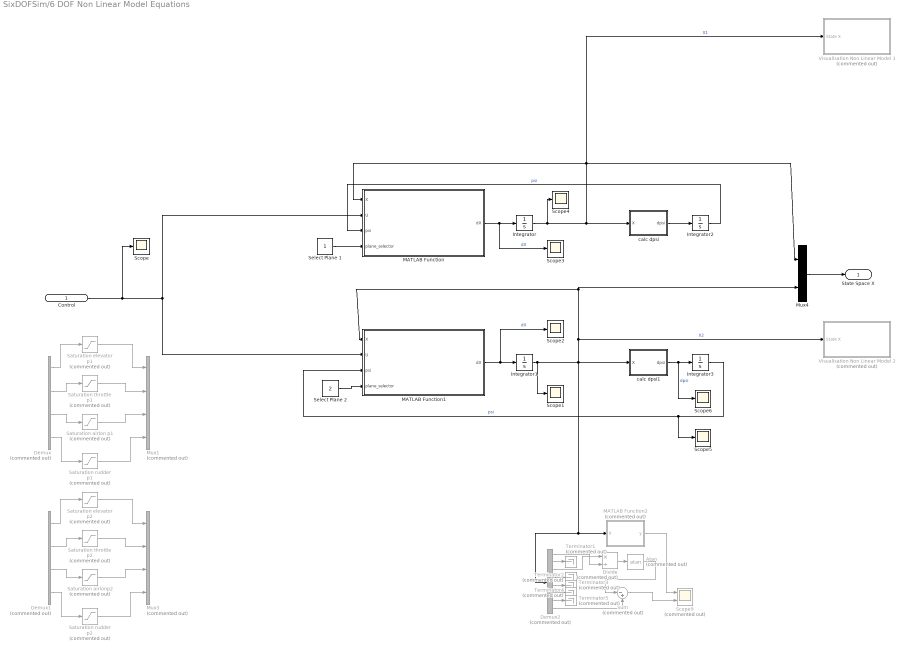
== system SixDOFSim/6 DOF Non Linear Model Equations ==
  Control : Inport
  Atan : Trigonometry  Commented=on  Operator=atan
  Demux : Demux  Commented=on
  Demux1 : Demux  Commented=on
  Demux2 : Demux  Commented=on  Outputs=8
  Divide : Product  Commented=on  Inputs=*/
  Integrator : Integrator  InitialCondition=X_ap_simulink(1:9)
  Integrator1 : Integrator  InitialCondition=X_ap_simulink(10:18)
  Integrator2 : Integrator
  Integrator3 : Integrator
  MATLAB Function : MATLAB Function  TreatAsAtomicUnit=on
  MATLAB Function1 : MATLAB Function  TreatAsAtomicUnit=on
  MATLAB Function2 : MATLAB Function  Commented=on  TreatAsAtomicUnit=on
  Mux1 : Mux  Commented=on
  Mux3 : Mux  Commented=on
  Mux4 : Mux  Inputs=2
  Saturation airlon p1 : Saturate  Commented=on  UpperLimit=xi_max  LowerLimit=xi_min
  Saturation airlonp2 : Saturate  Commented=on  UpperLimit=xi_max  LowerLimit=xi_min
  Saturation elevator p1 : Saturate  Commented=on  UpperLimit=eta_max  LowerLimit=eta_min
  Saturation elevator p2 : Saturate  Commented=on  UpperLimit=eta_max  LowerLimit=eta_min
  Saturation rudder p1 : Saturate  Commented=on  UpperLimit=zita_max  LowerLimit=zita_min
  Saturation rudder p2 : Saturate  Commented=on  UpperLimit=zita_max  LowerLimit=zita_min
  Saturation throttle p1 : Saturate  Commented=on  UpperLimit=sigmaf_max  LowerLimit=sigmaf_min
  Saturation throttle p2 : Saturate  Commented=on  UpperLimit=sigmaf_max  LowerLimit=sigmaf_min
  Scope{,1..6} (7 alike) : Scope
  Scope9 : Scope  Commented=on  NumInputPorts=2
  Select Plane 1 : Constant
  Select Plane 2 : Constant  Value=2
  Sum : Sum  Commented=on  Inputs=|-+
  Terminator{1..5} (5 alike) : Terminator  Commented=on
  Visualisation Non Linear Model 1 : Subsystem  Commented=on
  Visualisation Non Linear Model 2 : Subsystem  Commented=on
  calc dpsi : MATLAB Function  TreatAsAtomicUnit=on
  calc dpsi1 : MATLAB Function  TreatAsAtomicUnit=on
  State Space X : Outport
  wires:
  MATLAB Function/1(dX) -> Scope3/1, Integrator/1  "dX"
  Integrator/1 -> Scope4/1, MATLAB Function/1(X), Mux4/1, Visualisation Non Linear Model 1/1(State X), calc dpsi/1(X)  "X1"
  Demux/1 -> Saturation elevator p1/1
  Demux/2 -> Saturation throttle p1/1
  Demux/3 -> Saturation airlon p1/1
  Demux/4 -> Saturation rudder p1/1
  Saturation elevator p1/1 -> Mux1/1
  Saturation throttle p1/1 -> Mux1/2
  Saturation airlon p1/1 -> Mux1/3
  Saturation rudder p1/1 -> Mux1/4
  Integrator1/1 -> Demux2/1, MATLAB Function2/1(X), Mux4/2, MATLAB Function1/1(X), Visualisation Non Linear Model 2/1(State X), calc dpsi1/1(X), Scope1/1  "X2"
  Saturation rudder p2/1 -> Mux3/4
  Saturation throttle p2/1 -> Mux3/2
  Saturation elevator p2/1 -> Mux3/1
  Saturation airlonp2/1 -> Mux3/3
  Demux1/1 -> Saturation elevator p2/1
  Demux1/3 -> Saturation airlonp2/1
  Demux1/4 -> Saturation rudder p2/1
  Demux1/2 -> Saturation throttle p2/1
  MATLAB Function1/1(dX) -> Scope2/1, Integrator1/1  "dX"
  Control/1 -> MATLAB Function/2(U), MATLAB Function1/2(U), Scope/1
  Mux4/1 -> State Space X/1
  Select Plane 1/1 -> MATLAB Function/4(plane_selector)
  Select Plane 2/1 -> MATLAB Function1/4(plane_selector)
  calc dpsi/1(dpsi) -> Integrator2/1
  Integrator2/1 -> MATLAB Function/3(psi)  "psi"
  calc dpsi1/1(dpsi) -> Scope6/1, Integrator3/1  "dpsi"
  Integrator3/1 -> Scope5/1, MATLAB Function1/3(psi)  "psi"
  Demux2/8 -> Sum/2
  Demux2/3 -> Divide/1
  Demux2/1 -> Divide/2
  Demux2/2 -> Terminator1/1
  Demux2/4 -> Terminator2/1
  Demux2/5 -> Terminator3/1
  Demux2/6 -> Terminator4/1
  Demux2/7 -> Terminator5/1
  Divide/1 -> Atan/1
  Atan/1 -> Sum/1
  Sum/1 -> Scope9/2
  MATLAB Function2/1(y) -> Scope9/1

== system SixDOFSim/6 DOF Linear/Stellgrößenbeschränkung ==
  In1 : Inport
  Demux : Demux  Outputs=8
  Mux1 : Mux  Inputs=8
  Saturation airlon p1 : Saturate  UpperLimit=xi_max  LowerLimit=xi_min
  Saturation airlon p2 : Saturate  UpperLimit=xi_max  LowerLimit=xi_min
  Saturation elevator p1 : Saturate  UpperLimit=eta_max  LowerLimit=eta_min
  Saturation elevatorp2 : Saturate  UpperLimit=eta_max  LowerLimit=eta_min
  Saturation rudder p1 : Saturate  UpperLimit=zita_max  LowerLimit=zita_min
  Saturation rudder p2 : Saturate  UpperLimit=zita_max  LowerLimit=zita_min
  Saturation throttle p1 : Saturate  UpperLimit=sigmaf_max  LowerLimit=sigmaf_min
  Saturation throttle p2 : Saturate  UpperLimit=sigmaf_max  LowerLimit=sigmaf_min
  U_real : Outport
  wires:
  Demux/2 -> Saturation throttle p1/1
  Demux/3 -> Saturation airlon p1/1
  Demux/1 -> Saturation elevator p1/1
  Saturation airlon p2/1 -> Mux1/7
  Saturation rudder p1/1 -> Mux1/4
  Mux1/1 -> U_real/1  "U_real"
  Saturation airlon p1/1 -> Mux1/3
  Saturation elevator p1/1 -> Mux1/1
  Demux/4 -> Saturation rudder p1/1
  Saturation throttle p1/1 -> Mux1/2
  Saturation elevatorp2/1 -> Mux1/5
  Demux/8 -> Saturation rudder p2/1
  Demux/7 -> Saturation airlon p2/1
  Demux/6 -> Saturation throttle p2/1
  Saturation rudder p2/1 -> Mux1/8
  Demux/5 -> Saturation elevatorp2/1
  Saturation throttle p2/1 -> Mux1/6
  In1/1 -> Demux/1

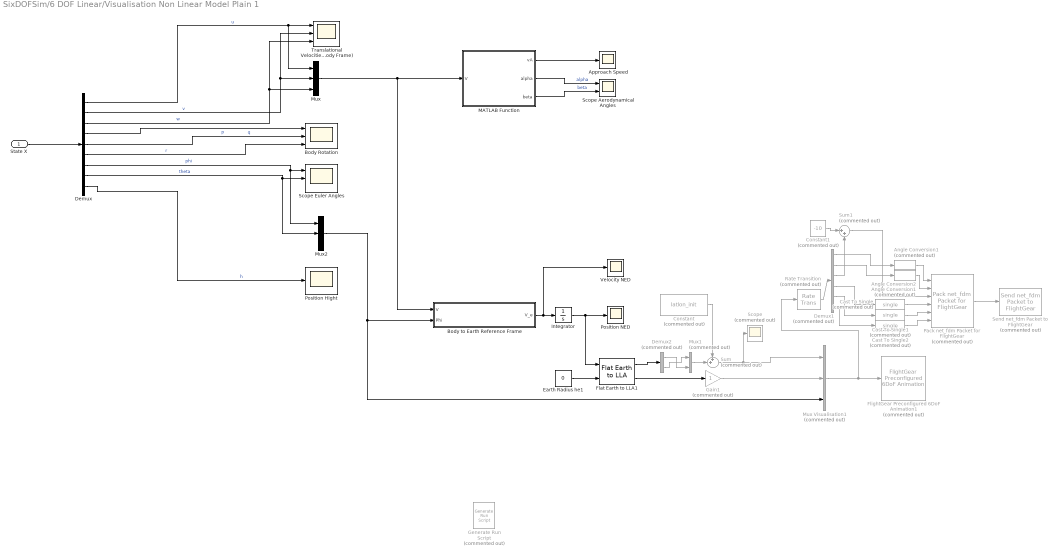
== system SixDOFSim/6 DOF Linear/Visualisation Non Linear Model Plain 1 ==
  State X : Inport
  Angle Conversion1 : aerolibfltsims/FlightGear Preconfigured 6DoF Animation/Angle Conversion1  Commented=on  SystemSampleTime=-1  VariantActivationTime=update diagram  Latency=0  AutoFrameSizeCalculation=off
      settings: SourceProductBaseCode=AE
  Angle Conversion2 : aerolibfltsims/FlightGear Preconfigured 6DoF Animation/Angle Conversion1  Commented=on  SystemSampleTime=-1  VariantActivationTime=update diagram  Latency=0  AutoFrameSizeCalculation=off
      settings: SourceProductBaseCode=AE
  Approach Speed : Scope
  Body Rotation : Scope  NumInputPorts=3
  "Body to Earth Reference Frame " : MATLAB Function  TreatAsAtomicUnit=on
  Cast To Single : DataTypeConversion  Commented=on  OutDataTypeStr=single
  Cast To Single1 : DataTypeConversion  Commented=on  OutDataTypeStr=single
  Cast To Single2 : DataTypeConversion  Commented=on  OutDataTypeStr=single
  Constant : Constant  Commented=on  Value=latlon_init
  Constant1 : Constant  Commented=on  Value=-10
  Demux : Demux  Outputs=9
  Demux1 : Demux  Commented=on  Outputs=6
  Demux2 : Demux  Commented=on  Outputs=2
  Earth Radius he1 : Constant  Value=0
  Flat Earth to LLA1 : aerolibtransform2/Flat Earth to LLA  units=Metric (MKS)  ptype=Earth (WGS84)  F=1/298.257223563  R=6378137  refPosPort=off  LL0=[0 10]  psi=0
  FlightGear Preconfigured 6DoF Animation1 : aerolibfltsims/FlightGear Preconfigured 6DoF Animation  Commented=on  xFlightGearVersion=v2019.1  DestinationIpAddress=127.0.0.1  DestinationPort=5502  SampleTime=1/30  packetVersion=24
  Gain1 : Gain  Commented=on
  Generate Run Script : aerolibfltsims/Generate Run Script  Commented=on  Architecture=Win64  dataFlow=Send  GeometryModelName=c172p  AirportId=KSFO  RunwayId=10L  InitialAltitude=7224  InitialHeading=113  OffsetDistance=4.72  OffsetAzimuth=0  InstallScenery=off  DisableShaders=on  OriginAddress=127.0.0.1  DestinationPort=5502  OriginPort=5505  LocalAddress=127.0.0.1  OutputFileName=runfg.bat  FlightGearBaseDirectory=D:\Flight Gear\FlightGear 2018.1.1
  Integrator : Integrator  InitialCondition=P_e_init_1
  MATLAB Function : MATLAB Function  TreatAsAtomicUnit=on
  Mux : Mux  Inputs=3
  Mux Visualisation1 : Mux  Commented=on  Inputs=3
  Mux1 : Mux  Commented=on  Inputs=2
  Mux2 : Mux  Inputs=3
  Pack net_fdm Packet for FlightGear : aerolibfltsims/Pack net_fdm Packet for FlightGear  Commented=on  FlightGearVersion=v2019.1  ShowPositionAttitudeInputs=on  ShowVelocityAccelerationInputs=off  ShowControlSurfacePositionInputs=off  ShowEngineFuelInputs=off  ShowLandingGearInputs=off  ShowEnvironmentInputs=off  SampleTime=1/30  packetVersion=24
      settings: SourceProductBaseCode=AE
  Position Hight : Scope
  Position NED : Scope
  Rate Transition : RateTransition  Commented=on  Integrity=off  Deterministic=off
  Scope : Scope  Commented=on
  Scope Aerodynamical Angles : Scope  NumInputPorts=2
  Scope Euler Angles : Scope  NumInputPorts=3
  Send net_fdm Packet to FlightGear : aerolibfltsims/Send net_fdm Packet to FlightGear  Commented=on  DestinationIpAddress=127.0.0.1  DestinationPort=5503  LocalIpPort=-1  varLen=off  SampleTime=1/30
      settings: SourceProductBaseCode=AE
  Sum : Sum  Commented=on  Inputs=++|
  Sum1 : Sum  Commented=on  Inputs=|++
  Translational Velocities (Body Frame) : Scope  NumInputPorts=3
  Velocity NED : Scope
  wires:
  State X/1 -> Demux/1
  Demux2/2 -> Mux1/1
  Flat Earth to LLA1/2 -> Gain1/1
  Gain1/1 -> Mux Visualisation1/2
  Mux Visualisation1/1 -> FlightGear Preconfigured 6DoF Animation1/1, Rate Transition/1
  Earth Radius he1/1 -> Flat Earth to LLA1/2
  Flat Earth to LLA1/1 -> Demux2/1
  Demux2/1 -> Mux1/2
  "Body to Earth Reference Frame "/1(V_e) -> Velocity NED/1, Integrator/1
  Integrator/1 -> Position NED/1, Flat Earth to LLA1/1
  Demux/1 -> Mux/1, Translational Velocities (Body Frame)/1  "u"
  Demux/2 -> Translational Velocities (Body Frame)/2, Mux/2  "v"
  Demux/3 -> Translational Velocities (Body Frame)/3, Mux/3  "w"
  Demux/4 -> Body Rotation/1  "p"
  Demux/5 -> Body Rotation/2  "q"
  Demux/6 -> Body Rotation/3  "r"
  Demux/7 -> Mux2/1, Scope Euler Angles/1  "phi"
  Demux/8 -> Mux2/2, Scope Euler Angles/2  "theta"
  Demux/9 -> Position Hight/1  "h"
  Mux/1 -> MATLAB Function/1(V), "Body to Earth Reference Frame "/1(V)
  Mux2/1 -> "Body to Earth Reference Frame "/2(Phi), Mux Visualisation1/3
  MATLAB Function/1(vA) -> Approach Speed/1
  MATLAB Function/2(alpha) -> Scope Aerodynamical Angles/1  "alpha"
  MATLAB Function/3(beta) -> Scope Aerodynamical Angles/2  "beta"
  Mux1/1 -> Sum/2
  Sum/1 -> Scope/1, Mux Visualisation1/1
  Constant/1 -> Sum/1
  Pack net_fdm Packet for FlightGear/1 -> Send net_fdm Packet to FlightGear/1
  Angle Conversion1/1 -> Pack net_fdm Packet for FlightGear/1
  Angle Conversion2/1 -> Pack net_fdm Packet for FlightGear/2
  Cast To Single/1 -> Pack net_fdm Packet for FlightGear/4
  Cast To Single1/1 -> Pack net_fdm Packet for FlightGear/5
  Cast To Single2/1 -> Pack net_fdm Packet for FlightGear/6
  Demux1/2 -> Angle Conversion2/1
  Rate Transition/1 -> Demux1/1
  Demux1/1 -> Angle Conversion1/1
  Constant1/1 -> Sum1/1
  Demux1/3 -> Sum1/2
  Sum1/1 -> Pack net_fdm Packet for FlightGear/3
  Demux1/4 -> Cast To Single/1
  Demux1/5 -> Cast To Single1/1
  Demux1/6 -> Cast To Single2/1

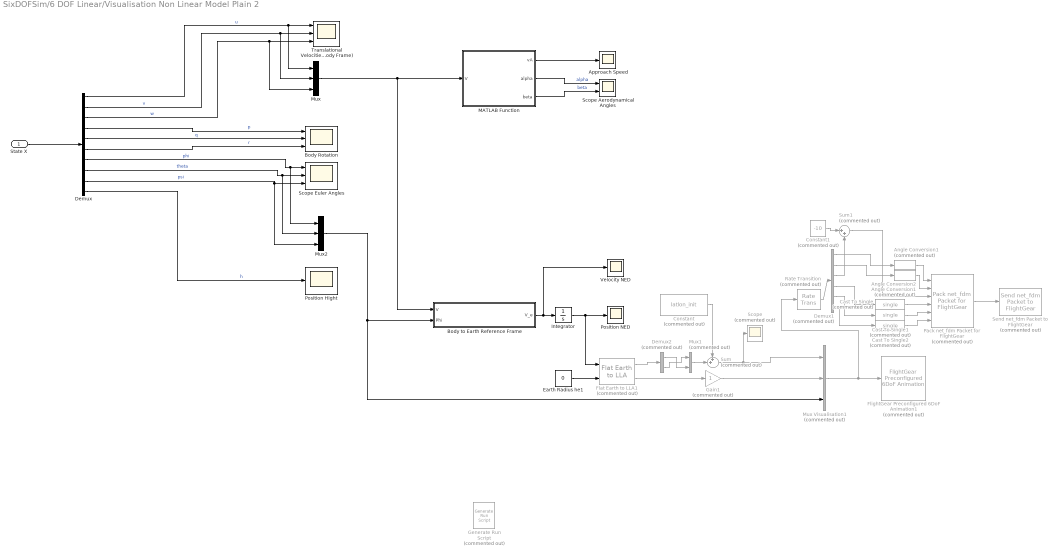
== system SixDOFSim/6 DOF Linear/Visualisation Non Linear Model Plain 2 ==
  State X : Inport
  Angle Conversion1 : aerolibfltsims/FlightGear Preconfigured 6DoF Animation/Angle Conversion1  Commented=on  SystemSampleTime=-1  VariantActivationTime=update diagram  Latency=0  AutoFrameSizeCalculation=off
      settings: SourceProductBaseCode=AE
  Angle Conversion2 : aerolibfltsims/FlightGear Preconfigured 6DoF Animation/Angle Conversion1  Commented=on  SystemSampleTime=-1  VariantActivationTime=update diagram  Latency=0  AutoFrameSizeCalculation=off
      settings: SourceProductBaseCode=AE
  Approach Speed : Scope
  Body Rotation : Scope  NumInputPorts=3
  "Body to Earth Reference Frame " : MATLAB Function  TreatAsAtomicUnit=on
  Cast To Single : DataTypeConversion  Commented=on  OutDataTypeStr=single
  Cast To Single1 : DataTypeConversion  Commented=on  OutDataTypeStr=single
  Cast To Single2 : DataTypeConversion  Commented=on  OutDataTypeStr=single
  Constant : Constant  Commented=on  Value=latlon_init
  Constant1 : Constant  Commented=on  Value=-10
  Demux : Demux  Outputs=10
  Demux1 : Demux  Commented=on  Outputs=6
  Demux2 : Demux  Commented=on  Outputs=2
  Earth Radius he1 : Constant  Value=0
  Flat Earth to LLA1 : aerolibtransform2/Flat Earth to LLA  Commented=on  units=Metric (MKS)  ptype=Earth (WGS84)  F=1/298.257223563  R=6378137  refPosPort=off  LL0=[0 10]  psi=0
  FlightGear Preconfigured 6DoF Animation1 : aerolibfltsims/FlightGear Preconfigured 6DoF Animation  Commented=on  xFlightGearVersion=v2019.1  DestinationIpAddress=127.0.0.1  DestinationPort=5502  SampleTime=1/30  packetVersion=24
  Gain1 : Gain  Commented=on
  Generate Run Script : aerolibfltsims/Generate Run Script  Commented=on  Architecture=Win64  dataFlow=Send  GeometryModelName=c172p  AirportId=KSFO  RunwayId=10L  InitialAltitude=7224  InitialHeading=113  OffsetDistance=4.72  OffsetAzimuth=0  InstallScenery=off  DisableShaders=on  OriginAddress=127.0.0.1  DestinationPort=5502  OriginPort=5505  LocalAddress=127.0.0.1  OutputFileName=runfg.bat  FlightGearBaseDirectory=D:\Flight Gear\FlightGear 2018.1.1
  Integrator : Integrator  InitialCondition=P_e_init_2
  MATLAB Function : MATLAB Function  TreatAsAtomicUnit=on
  Mux : Mux  Inputs=3
  Mux Visualisation1 : Mux  Commented=on  Inputs=3
  Mux1 : Mux  Commented=on  Inputs=2
  Mux2 : Mux  Inputs=3
  Pack net_fdm Packet for FlightGear : aerolibfltsims/Pack net_fdm Packet for FlightGear  Commented=on  FlightGearVersion=v2019.1  ShowPositionAttitudeInputs=on  ShowVelocityAccelerationInputs=off  ShowControlSurfacePositionInputs=off  ShowEngineFuelInputs=off  ShowLandingGearInputs=off  ShowEnvironmentInputs=off  SampleTime=1/30  packetVersion=24
      settings: SourceProductBaseCode=AE
  Position Hight : Scope
  Position NED : Scope
  Rate Transition : RateTransition  Commented=on  Integrity=off  Deterministic=off
  Scope : Scope  Commented=on
  Scope Aerodynamical Angles : Scope  NumInputPorts=2
  Scope Euler Angles : Scope  NumInputPorts=3
  Send net_fdm Packet to FlightGear : aerolibfltsims/Send net_fdm Packet to FlightGear  Commented=on  DestinationIpAddress=127.0.0.1  DestinationPort=5503  LocalIpPort=-1  varLen=off  SampleTime=1/30
      settings: SourceProductBaseCode=AE
  Sum : Sum  Commented=on  Inputs=++|
  Sum1 : Sum  Commented=on  Inputs=|++
  Translational Velocities (Body Frame) : Scope  NumInputPorts=3
  Velocity NED : Scope
  wires:
  State X/1 -> Demux/1
  Demux2/2 -> Mux1/1
  Flat Earth to LLA1/2 -> Gain1/1
  Gain1/1 -> Mux Visualisation1/2
  Mux Visualisation1/1 -> FlightGear Preconfigured 6DoF Animation1/1, Rate Transition/1
  Earth Radius he1/1 -> Flat Earth to LLA1/2
  Flat Earth to LLA1/1 -> Demux2/1
  Demux2/1 -> Mux1/2
  "Body to Earth Reference Frame "/1(V_e) -> Velocity NED/1, Integrator/1
  Integrator/1 -> Position NED/1, Flat Earth to LLA1/1
  Demux/1 -> Mux/1, Translational Velocities (Body Frame)/1  "u"
  Demux/2 -> Mux/2, Translational Velocities (Body Frame)/2  "v"
  Demux/3 -> Translational Velocities (Body Frame)/3, Mux/3  "w"
  Demux/4 -> Body Rotation/1  "p"
  Demux/5 -> Body Rotation/2  "q"
  Demux/6 -> Body Rotation/3  "r"
  Demux/7 -> Mux2/1, Scope Euler Angles/1  "phi"
  Demux/8 -> Mux2/2, Scope Euler Angles/2  "theta"
  Demux/9 -> Mux2/3, Scope Euler Angles/3  "psi"
  Demux/10 -> Position Hight/1  "h"
  Mux/1 -> MATLAB Function/1(V), "Body to Earth Reference Frame "/1(V)
  Mux2/1 -> "Body to Earth Reference Frame "/2(Phi), Mux Visualisation1/3
  MATLAB Function/1(vA) -> Approach Speed/1
  MATLAB Function/2(alpha) -> Scope Aerodynamical Angles/1  "alpha"
  MATLAB Function/3(beta) -> Scope Aerodynamical Angles/2  "beta"
  Mux1/1 -> Sum/2
  Sum/1 -> Scope/1, Mux Visualisation1/1
  Constant/1 -> Sum/1
  Pack net_fdm Packet for FlightGear/1 -> Send net_fdm Packet to FlightGear/1
  Angle Conversion1/1 -> Pack net_fdm Packet for FlightGear/1
  Angle Conversion2/1 -> Pack net_fdm Packet for FlightGear/2
  Cast To Single/1 -> Pack net_fdm Packet for FlightGear/4
  Cast To Single1/1 -> Pack net_fdm Packet for FlightGear/5
  Cast To Single2/1 -> Pack net_fdm Packet for FlightGear/6
  Demux1/2 -> Angle Conversion2/1
  Rate Transition/1 -> Demux1/1
  Demux1/1 -> Angle Conversion1/1
  Constant1/1 -> Sum1/1
  Demux1/3 -> Sum1/2
  Sum1/1 -> Pack net_fdm Packet for FlightGear/3
  Demux1/4 -> Cast To Single/1
  Demux1/5 -> Cast To Single1/1
  Demux1/6 -> Cast To Single2/1

== system SixDOFSim/6 DOF Model Boeing 757 200/Forces and Moments Plane 2 ==
  Throttel Position sigmaf : Inport
  Approach speed vA : Inport  Port=2
  Angle of Attack Alpha : Inport  Port=3
  Slide Angle  beta : Inport  Port=4
  Lift Coeficcient CA : Inport  Port=5
  Drag Coefficient CW : Inport  Port=6
  Sideforce Coefficient CQ : Inport  Port=7
  CL : Inport  Port=8
  CM : Inport  Port=9
  CN : Inport  Port=10
  Air Density rho : Inport  Port=11
  Aerodynamical Forces : MATLAB Function  TreatAsAtomicUnit=on
  Aerodynamical Forces RA Plane 1 : Scope
  Aerodynamical Torque : MATLAB Function  TreatAsAtomicUnit=on
  Aerodynamical Torque QA Plane 1 : Scope
  Sum : Sum  Inputs=++|
  Sum1 : Sum  Inputs=|++
  Thrust Force and Torque : MATLAB Function  TreatAsAtomicUnit=on
  Sum of external Forces : Outport
  Sum of external Torques : Outport  Port=2
  wires:
  Air Density rho/1 -> Aerodynamical Torque/6(rho), Aerodynamical Forces/7(rho)
  CN/1 -> Aerodynamical Torque/4(CN)
  CM/1 -> Aerodynamical Torque/3(CM)
  CL/1 -> Aerodynamical Torque/2(CL)
  Sideforce Coefficient CQ/1 -> Aerodynamical Forces/3(CQ)
  Drag Coefficient CW/1 -> Aerodynamical Forces/2(CW)
  Lift Coeficcient CA/1 -> Aerodynamical Forces/1(CA)
  Approach speed vA/1 -> Aerodynamical Torque/5(vA), Aerodynamical Forces/4(vA)
  Slide Angle  beta/1 -> Aerodynamical Forces/6(beta)
  Angle of Attack Alpha/1 -> Aerodynamical Forces/5(alpha)
  Thrust Force and Torque/2(Qf) -> Sum/1
  Thrust Force and Torque/1(Rf) -> Sum1/2
  Throttel Position sigmaf/1 -> Thrust Force and Torque/1(sigmaf)
  Sum/1 -> Sum of external Torques/1
  Sum1/1 -> Sum of external Forces/1
  Aerodynamical Torque/1(QA) -> Aerodynamical Torque QA Plane 1/1, Sum/2
  Aerodynamical Forces/1(RA) -> Aerodynamical Torque/1(RA), Sum1/1, Aerodynamical Forces RA Plane 1/1

== system SixDOFSim/6 DOF Model Boeing 757 200/Forces and Moments Plane 3 ==
  Throttel Position sigmaf : Inport
  Approach speed vA : Inport  Port=2
  Angle of Attack Alpha : Inport  Port=3
  Slide Angle  beta : Inport  Port=4
  Lift Coeficcient CA : Inport  Port=5
  Drag Coefficient CW : Inport  Port=6
  Sideforce Coefficient CQ : Inport  Port=7
  CL : Inport  Port=8
  CM : Inport  Port=9
  CN : Inport  Port=10
  Air Density rho : Inport  Port=11
  Aerodynamical Forces : MATLAB Function  TreatAsAtomicUnit=on
  Aerodynamical Forces RA Plane 2 : Scope
  Aerodynamical Torque : MATLAB Function  TreatAsAtomicUnit=on
  Aerodynamical Torque QA Plane 2 : Scope
  Sum : Sum  Inputs=++|
  Sum1 : Sum  Inputs=|++
  Thrust Force and Torque : MATLAB Function  TreatAsAtomicUnit=on
  Sum of external Forces : Outport
  Sum of external Torques : Outport  Port=2
  wires:
  Aerodynamical Forces/1(RA) -> Aerodynamical Forces RA Plane 2/1, Sum1/1, Aerodynamical Torque/1(RA)
  Aerodynamical Torque/1(QA) -> Sum/2, Aerodynamical Torque QA Plane 2/1
  Sum1/1 -> Sum of external Forces/1
  Sum/1 -> Sum of external Torques/1
  Throttel Position sigmaf/1 -> Thrust Force and Torque/1(sigmaf)
  Thrust Force and Torque/1(Rf) -> Sum1/2
  Thrust Force and Torque/2(Qf) -> Sum/1
  Angle of Attack Alpha/1 -> Aerodynamical Forces/5(alpha)
  Slide Angle  beta/1 -> Aerodynamical Forces/6(beta)
  Approach speed vA/1 -> Aerodynamical Forces/4(vA), Aerodynamical Torque/5(vA)
  Lift Coeficcient CA/1 -> Aerodynamical Forces/1(CA)
  Drag Coefficient CW/1 -> Aerodynamical Forces/2(CW)
  Sideforce Coefficient CQ/1 -> Aerodynamical Forces/3(CQ)
  CL/1 -> Aerodynamical Torque/2(CL)
  CM/1 -> Aerodynamical Torque/3(CM)
  CN/1 -> Aerodynamical Torque/4(CN)
  Air Density rho/1 -> Aerodynamical Forces/7(rho), Aerodynamical Torque/6(rho)
